simulink model "DOB"  (R2023a)
settings: Solver=VariableStepAuto  StartTime=0.0  StopTime=50  RelTol=1e-3
values from neighbouring files (symbols this model uses):
  K = lqr(sys, Q, R)    [lqrController.m]
settings Model: Creator=belov  LastModifiedBy=belov

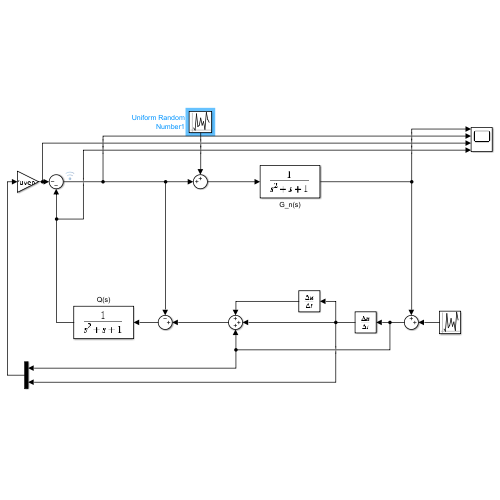
[thumbnail: Simulink's stored preview of the top-level diagram]
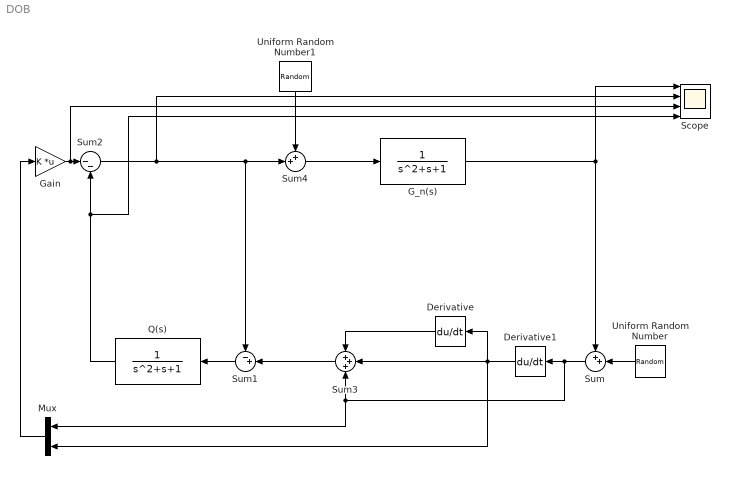
== system DOB ==
  Derivative : Derivative
  Derivative1 : Derivative
  G_n(s) : TransferFcn  Denominator=[1 1 1]
  Gain : Gain  Gain=K  Multiplication=Matrix(K*u) (u vector)
  Mux : Mux  Inputs=2
  Q(s) : TransferFcn  Denominator=[1 1 1]
  Scope : Scope  NumInputPorts=4
  Sum : Sum  Inputs=++|
  Sum1 : Sum  Inputs=-+|
  Sum2 : Sum  Inputs=|--
  Sum3 : Sum  Inputs=+++
  Sum4 : Sum  Inputs=++|
  Uniform Random Number : UniformRandomNumber  Minimum=-0.02  Maximum=0.02  SampleTime=0.001
  Uniform Random Number1 : UniformRandomNumber  Minimum=-0.05  Maximum=0.05  SampleTime=0.001
  wires:
  G_n(s)/1 -> Scope/1, Sum/1
  Sum/1 -> Mux/1, Sum3/3, Derivative1/1
  Sum2/1 -> Scope/2, Sum1/1, Sum4/2
  Sum3/1 -> Sum1/2
  Sum1/1 -> Q(s)/1
  Derivative/1 -> Sum3/1
  Derivative1/1 -> Mux/2, Sum3/2, Derivative/1
  Gain/1 -> Scope/3, Sum2/1
  Mux/1 -> Gain/1
  Sum4/1 -> G_n(s)/1
  Uniform Random Number1/1 -> Sum4/1
  Uniform Random Number/1 -> Sum/2
  Q(s)/1 -> Scope/4, Sum2/2
